simulink model "test_3Lpwm"  (R2025b)
settings: Solver=ode23tb  StartTime=0.0  StopTime=0.2  FixedStep=tc  MaxStep=tc
undefined symbols (not defined in the file or in its folder): dead_time_INV, fPWM_INV, tc, ts_afe
libraries: eePwmGeneratorThreeLevel x1, single_phase_pwm_modulator x1
settings Model: SimulationMode=accelerator  Creator=dbagn  LastModifiedBy=dbagn
settings SolverCC: NumberNewtonIterations=3.0  ZeroCrossControl=DisableAll  AlgebraicLoopSolver=TrustRegion  SolverResetMethod=Robust
settings DataIOCC: ReturnWorkspaceOutputs=off
settings OptimizationCC: ReuseModelBlockBuffer=off
settings DebuggingCC: UnconnectedInputMsg=warning  UnconnectedOutputMsg=warning  UnconnectedLineMsg=warning
settings ModelReferenceCC: EnableRefExpFcnMdlSchedulingChecks=on
settings SFSimCC: CustomCodeUndefinedFunction=ThrowError
settings SFSimCC: SimCustomHeaderCode=|
  | #include "mavgflt.h"
  | #include "mavgflt_simulink.h"
  | #include "bemf_obsv.h"
  | #include "bemf_obsv_simulink.h"
  | #include "bemf_obsv_load_est.h"
  | #include "bemf_obsv_load_est_simulink.h"
  | #include "dqvector_pi.h"
  | #include "dqvector_pi_simulink.h"
  | #include "sv_pwm_simulink.h"
  | #include "sv_pwm.h"
  | #include "first_harmonic_tracker.h"
  | #include "first_harmonic_tracker_simulink.h"
  | #include "dqpll_thyr.h"
  | #include "dqpll_thyr_simulink.h"
  | #include "dqpll_grid.h"
  | #include "dqpll_grid_simulink.h"
settings SFSimCC: SimUserSources=|
  | "mavgflt_simulink.c"
  | "mavgflt.c"
  | "bemf_obsv_simulink.c"
  | "bemf_obsv.c"
  | "bemf_obsv_load_est_simulink.c"
  | "bemf_obsv_load_est.c"
  | "dqvector_pi.c"
  | "dqvector_pi_simulink.c"
  | "sv_pwm_simulink.c"
  | "sv_pwm.c"
  | "first_harmonic_tracker_simulink.c"
  | "first_harmonic_tracker.c"
  | "dqpll_thyr_simulink.c"
  | "dqpll_thyr.c"
  | "dqpll_grid_simulink.c"
  | "dqpll_grid.c"
settings SFSimCC: SimUserIncludeDirs=|
  | include
  | src
settings RTWCC: GPUComputeCapability=3.5  DLArmComputeVersion=19.05

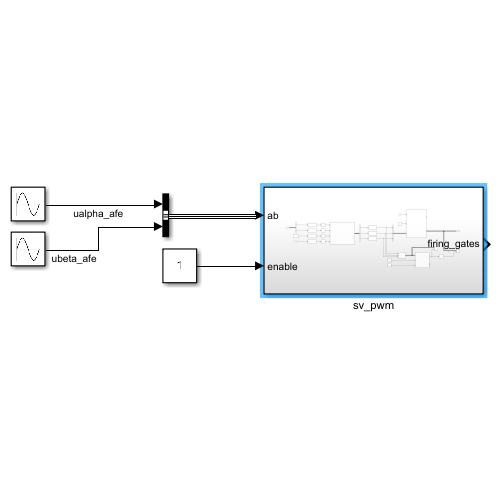
[thumbnail: Simulink's stored preview of the top-level diagram]
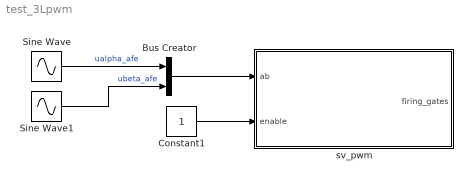
== system test_3Lpwm ==
  Bus Creator : BusCreator  Inputs=2
  Constant1 : Constant
  Sine Wave : Sin  Amplitude=sqrt(3)/2  Frequency=2*pi*50  Phase=-pi/2  SampleTime=0
  Sine Wave1 : Sin  Amplitude=sqrt(3)/2  Frequency=2*pi*50  SampleTime=0
  sv_pwm : Subsystem
  wires:
  Constant1/1 -> sv_pwm/2(enable)
  Bus Creator/1 -> sv_pwm/1(ab)
  Sine Wave/1 -> Bus Creator/1  "ualpha_afe"
  Sine Wave1/1 -> Bus Creator/2  "ubeta_afe"

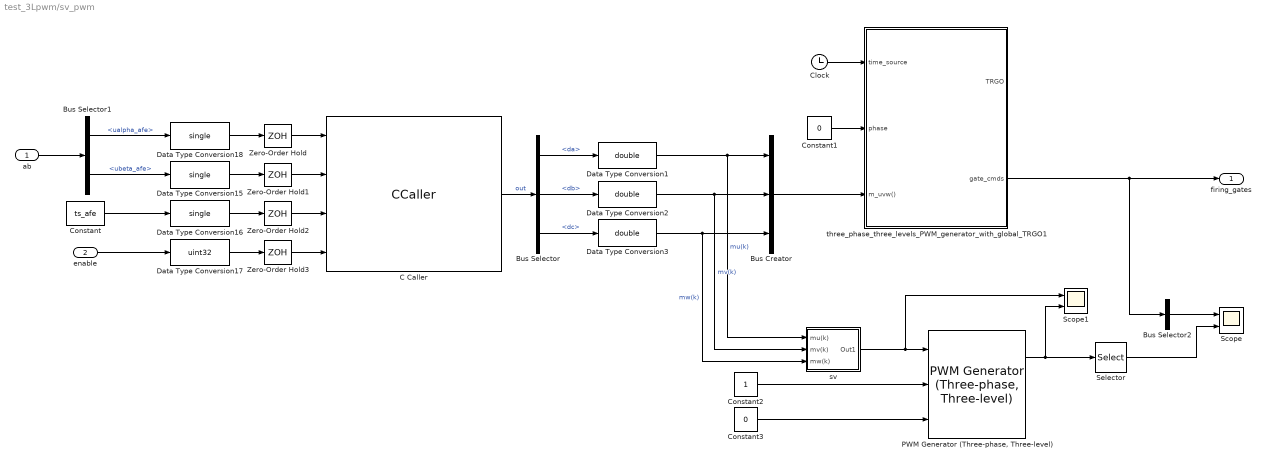
== system test_3Lpwm/sv_pwm ==
  ab : Inport
  enable : Inport  Port=2
  Bus Creator : BusCreator  Inputs=3
  Bus Selector : BusSelector  OutputSignals=da,db,dc
  Bus Selector1 : BusSelector  OutputSignals=ualpha_afe,ubeta_afe
  Bus Selector2 : BusSelector  OutputSignals=gate_cmds_phu  OutputAsBus=on
  C Caller : CCaller  FunctionName=sv_pwm_process_simulink  PortSpecificationStruct="%)30     .    V @   8    (     @         %    \"     4    !     0         %  0 \"0    $    _    07)G3F%M90  4&]R=$YA;64 4V-O<&4     26YD97@     5'EP90      4VEZ90      27-';&]B86P   X    P    !@    @    $          4    (     0    ,    !         !   P!O=70 #@   #     &    \"     0         !0    @    !     P    $         $  # &]U=  .    .     8    (    !          %    \"     $    &     0         0   ...(+2669 chars)"  SampleTime=ts_afe
  Clock : Clock
  Constant : Constant  Value=ts_afe
  Constant1 : Constant  Value=0
  Constant2 : Constant
  Constant3 : Constant  Value=0
  Data Type Conversion1 : DataTypeConversion  OutDataTypeStr=double  SaturateOnIntegerOverflow=off  RndMeth=Floor
  Data Type Conversion15 : DataTypeConversion  OutDataTypeStr=single  SaturateOnIntegerOverflow=off  RndMeth=Floor
  Data Type Conversion16 : DataTypeConversion  OutDataTypeStr=single  SaturateOnIntegerOverflow=off  RndMeth=Floor
  Data Type Conversion17 : DataTypeConversion  OutDataTypeStr=uint32  SaturateOnIntegerOverflow=off  RndMeth=Floor
  Data Type Conversion18 : DataTypeConversion  OutDataTypeStr=single  SaturateOnIntegerOverflow=off  RndMeth=Floor
  Data Type Conversion2 : DataTypeConversion  OutDataTypeStr=double  SaturateOnIntegerOverflow=off  RndMeth=Floor
  Data Type Conversion3 : DataTypeConversion  OutDataTypeStr=double  SaturateOnIntegerOverflow=off  RndMeth=Floor
  "PWM Generator (Three-phase, Three-level)" : eePwmGeneratorThreeLevel/PWM Generator (Three-phase, Three-level)  CPWMMode=SPWM: sinusoidal PWM  fsw=1e3  Ts=5e-5
      settings: SamplingMode=Natural
      settings: LibrarySourceBlock=|
      | ee_sl_lib/Pulse Width
      | Modulation/PWM Generator
      | (Three-phase, Three-level)
  Scope : Scope  NumInputPorts=2
      settings: ActiveDisplayYMinimum=-13.125  ActiveDisplayYMaximum=18.125  DataLoggingVariableName=ScopeData6
  Scope1 : Scope  NumInputPorts=2
      settings: ActiveDisplayYMinimum=-2.2498929426074028  ActiveDisplayYMaximum=0.24989300221204752
  Selector : Selector  InputPortWidth=12  IndexOptions=Index vector (dialog)  Indices=[1 2 3 4]  OutputSizes=1
  Zero-Order Hold{,1..3} (4 alike) : ZeroOrderHold  SampleTime=ts_afe
  sv : Subsystem
  three_phase_three_levels_PWM_generator_with_global_TRGO1 : Subsystem  mask{f=fPWM_INV, m_up=1, m_low=-1, dead_time=dead_time_INV, pos_cmd_gate=15, neg_cmd_gate=-10, polarity=1, tc=tc, double_sampling=1}
      mask prompts: f "Frequency (Hz)"; m_up "Max Input Modulation Value"; m_low "Min Input Modulation Value"; dead_time "Dead Time (s)"; pos_cmd_gate "Positive Gate Voltage (V)"; neg_cmd_gate "Negative Gate Voltage (V)"; polarity "Polarity (pu)"; tc "Sampling time"; double_sampling "double TRGO update"
  firing_gates : Outport
  wires:
  Zero-Order Hold2/1 -> C Caller/3
  Constant/1 -> Data Type Conversion16/1
  Data Type Conversion18/1 -> Zero-Order Hold/1
  enable/1 -> Data Type Conversion17/1
  Data Type Conversion16/1 -> Zero-Order Hold2/1
  Data Type Conversion17/1 -> Zero-Order Hold3/1
  Zero-Order Hold3/1 -> C Caller/4
  Data Type Conversion15/1 -> Zero-Order Hold1/1
  three_phase_three_levels_PWM_generator_with_global_TRGO1/2(gate_cmds) -> Bus Selector2/1, firing_gates/1
  Bus Selector1/1 -> Data Type Conversion18/1  "<ualpha_afe>"
  Bus Selector1/2 -> Data Type Conversion15/1  "<ubeta_afe>"
  Data Type Conversion3/1 -> sv/3(mw(k)), Bus Creator/3  "mw(k)"
  Data Type Conversion2/1 -> sv/2(mv(k)), Bus Creator/2  "mv(k)"
  Data Type Conversion1/1 -> sv/1(mu(k)), Bus Creator/1  "mu(k)"
  ab/1 -> Bus Selector1/1
  Zero-Order Hold/1 -> C Caller/1
  Zero-Order Hold1/1 -> C Caller/2
  C Caller/1 -> Bus Selector/1  "out"
  Bus Selector/1 -> Data Type Conversion1/1  "<da>"
  Bus Selector/2 -> Data Type Conversion2/1  "<db>"
  Bus Selector/3 -> Data Type Conversion3/1  "<dc>"
  Clock/1 -> three_phase_three_levels_PWM_generator_with_global_TRGO1/1(time_source)
  Bus Creator/1 -> three_phase_three_levels_PWM_generator_with_global_TRGO1/3(m_uvw())
  Constant1/1 -> three_phase_three_levels_PWM_generator_with_global_TRGO1/2(phase)
  Bus Selector2/1 -> Scope/1
  Constant2/1 -> "PWM Generator (Three-phase, Three-level)"/2
  Constant3/1 -> "PWM Generator (Three-phase, Three-level)"/3
  "PWM Generator (Three-phase, Three-level)"/1 -> Scope1/2, Selector/1
  Selector/1 -> Scope/2
  sv/1(Out1) -> Scope1/1, "PWM Generator (Three-phase, Three-level)"/1

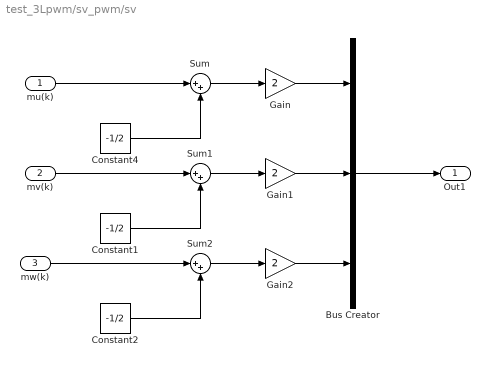
== system test_3Lpwm/sv_pwm/sv ==
  mu(k) : Inport
  mv(k) : Inport  Port=2
  mw(k) : Inport  Port=3
  Bus Creator : BusCreator  Inputs=3
  Constant1 : Constant  Value=-1/2
  Constant2 : Constant  Value=-1/2
  Constant4 : Constant  Value=-1/2
  Gain : Gain  Gain=2
  Gain1 : Gain  Gain=2
  Gain2 : Gain  Gain=2
  Sum : Sum  Inputs=|++
  Sum1 : Sum  Inputs=|++
  Sum2 : Sum  Inputs=|++
  Out1 : Outport
  wires:
  Sum/1 -> Gain/1
  mu(k)/1 -> Sum/1
  Constant4/1 -> Sum/2
  Gain/1 -> Bus Creator/1
  Bus Creator/1 -> Out1/1
  Constant1/1 -> Sum1/2
  Sum1/1 -> Gain1/1
  Gain1/1 -> Bus Creator/2
  mv(k)/1 -> Sum1/1
  mw(k)/1 -> Sum2/1
  Sum2/1 -> Gain2/1
  Constant2/1 -> Sum2/2
  Gain2/1 -> Bus Creator/3

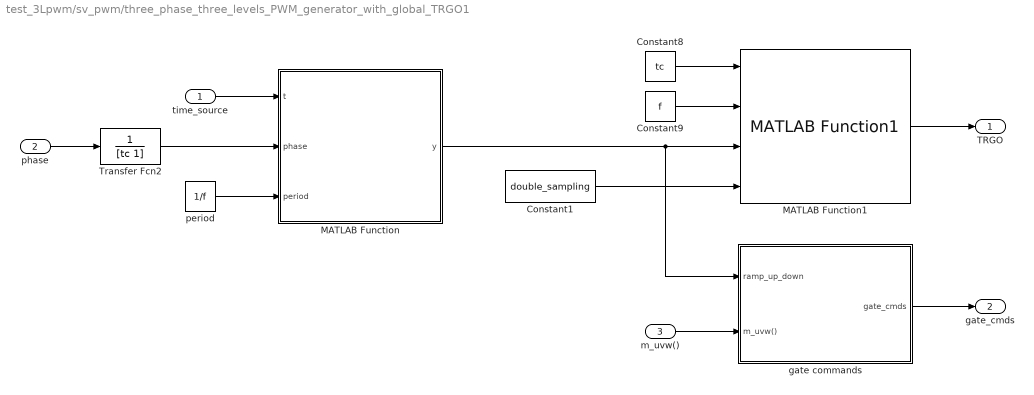
== system test_3Lpwm/sv_pwm/three_phase_three_levels_PWM_generator_with_global_TRGO1 ==
  time_source : Inport
  phase : Inport  Port=2
  m_uvw() : Inport  Port=3
  Constant1 : Constant  Value=double_sampling
  Constant8 : Constant  Value=tc
  Constant9 : Constant  Value=f
  MATLAB Function : MATLAB Function  TreatAsAtomicUnit=on  SystemSampleTime=tc
  MATLAB Function1 : single_phase_pwm_modulator/Single phase two level PWM generator with global TRGO/MATLAB Function1  SystemSampleTime=tc  VariantActivationTime=update diagram  EmptyChoice=off  PassThrough=off  PassThroughVariantControl=(default)  EmptyChoiceVariantControl=(default)  AllowFlexibleInterface=on  Latency=0  AutoFrameSizeCalculation=off
  Transfer Fcn2 : TransferFcn  Denominator=[tc 1]
  gate commands : Subsystem
  period : Constant  Value=1/f
  TRGO : Outport
  gate_cmds : Outport  Port=2
  wires:
  Transfer Fcn2/1 -> MATLAB Function/2(phase)
  Constant1/1 -> MATLAB Function1/4
  time_source/1 -> MATLAB Function/1(t)
  gate commands/1(gate_cmds) -> gate_cmds/1
  m_uvw()/1 -> gate commands/2(m_uvw())
  Constant9/1 -> MATLAB Function1/2
  Constant8/1 -> MATLAB Function1/1
  MATLAB Function1/1 -> TRGO/1
  MATLAB Function/1(y) -> MATLAB Function1/3, gate commands/1(ramp_up_down)
  phase/1 -> Transfer Fcn2/1
  period/1 -> MATLAB Function/3(period)

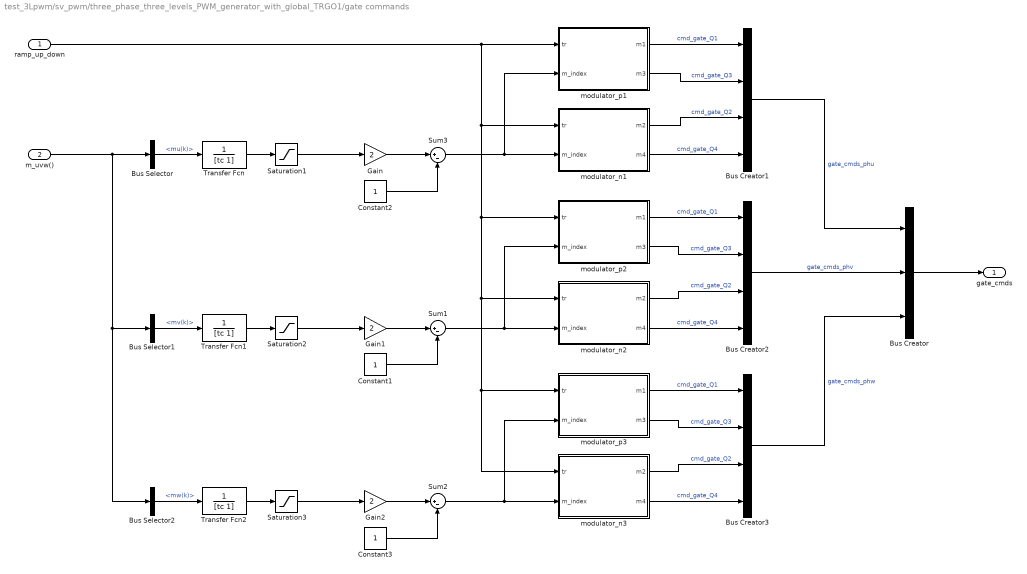
== system test_3Lpwm/sv_pwm/three_phase_three_levels_PWM_generator_with_global_TRGO1/gate commands ==
  ramp_up_down : Inport
  m_uvw() : Inport  Port=2
  Bus Creator : BusCreator  Inputs=3
  Bus Creator1 : BusCreator  Inputs=4
  Bus Creator2 : BusCreator  Inputs=4
  Bus Creator3 : BusCreator  Inputs=4
  Bus Selector : BusSelector  OutputSignals=mu(k)
  Bus Selector1 : BusSelector  OutputSignals=mv(k)
  Bus Selector2 : BusSelector  OutputSignals=mw(k)
  Constant1 : Constant
  Constant2 : Constant
  Constant3 : Constant
  Gain : Gain  Gain=2
  Gain1 : Gain  Gain=2
  Gain2 : Gain  Gain=2
  Saturation1 : Saturate  UpperLimit=m_up  LowerLimit=m_low
  Saturation2 : Saturate  UpperLimit=m_up  LowerLimit=m_low
  Saturation3 : Saturate  UpperLimit=m_up  LowerLimit=m_low
  Sum1 : Sum  Inputs=|+-
  Sum2 : Sum  Inputs=|+-
  Sum3 : Sum  Inputs=|+-
  Transfer Fcn : TransferFcn  Denominator=[tc 1]
  Transfer Fcn1 : TransferFcn  Denominator=[tc 1]
  Transfer Fcn2 : TransferFcn  Denominator=[tc 1]
  modulator_n1 : Subsystem
  modulator_n2 : Subsystem
  modulator_n3 : Subsystem
  modulator_p1 : Subsystem
  modulator_p2 : Subsystem
  modulator_p3 : Subsystem
  gate_cmds : Outport
  wires:
  Transfer Fcn2/1 -> Saturation3/1
  Transfer Fcn1/1 -> Saturation2/1
  Transfer Fcn/1 -> Saturation1/1
  Bus Selector/1 -> Transfer Fcn/1  "<mu(k)>"
  Bus Selector2/1 -> Transfer Fcn2/1  "<mw(k)>"
  Bus Selector1/1 -> Transfer Fcn1/1  "<mv(k)>"
  Bus Creator/1 -> gate_cmds/1
  m_uvw()/1 -> Bus Selector/1, Bus Selector1/1, Bus Selector2/1
  Gain/1 -> Sum3/1
  Sum3/1 -> modulator_p1/2(m_index), modulator_n1/2(m_index)
  Constant2/1 -> Sum3/2
  Saturation1/1 -> Gain/1
  modulator_p1/1(m1) -> Bus Creator1/1  "cmd_gate_Q1"
  modulator_p1/2(m3) -> Bus Creator1/2  "cmd_gate_Q3"
  modulator_n1/1(m2) -> Bus Creator1/3  "cmd_gate_Q2"
  modulator_n1/2(m4) -> Bus Creator1/4  "cmd_gate_Q4"
  Bus Creator1/1 -> Bus Creator/1  "gate_cmds_phu"
  Bus Creator2/1 -> Bus Creator/2  "gate_cmds_phv"
  modulator_n2/2(m4) -> Bus Creator2/4  "cmd_gate_Q4"
  modulator_n2/1(m2) -> Bus Creator2/3  "cmd_gate_Q2"
  modulator_p2/2(m3) -> Bus Creator2/2  "cmd_gate_Q3"
  modulator_p2/1(m1) -> Bus Creator2/1  "cmd_gate_Q1"
  ramp_up_down/1 -> modulator_n2/1(tr), modulator_p3/1(tr), modulator_n3/1(tr), modulator_p2/1(tr), modulator_n1/1(tr), modulator_p1/1(tr)
  modulator_p3/1(m1) -> Bus Creator3/1  "cmd_gate_Q1"
  modulator_p3/2(m3) -> Bus Creator3/2  "cmd_gate_Q3"
  modulator_n3/1(m2) -> Bus Creator3/3  "cmd_gate_Q2"
  modulator_n3/2(m4) -> Bus Creator3/4  "cmd_gate_Q4"
  Bus Creator3/1 -> Bus Creator/3  "gate_cmds_phw"
  Constant1/1 -> Sum1/2
  Gain1/1 -> Sum1/1
  Saturation2/1 -> Gain1/1
  Sum1/1 -> modulator_p2/2(m_index), modulator_n2/2(m_index)
  Sum2/1 -> modulator_n3/2(m_index), modulator_p3/2(m_index)
  Saturation3/1 -> Gain2/1
  Gain2/1 -> Sum2/1
  Constant3/1 -> Sum2/2

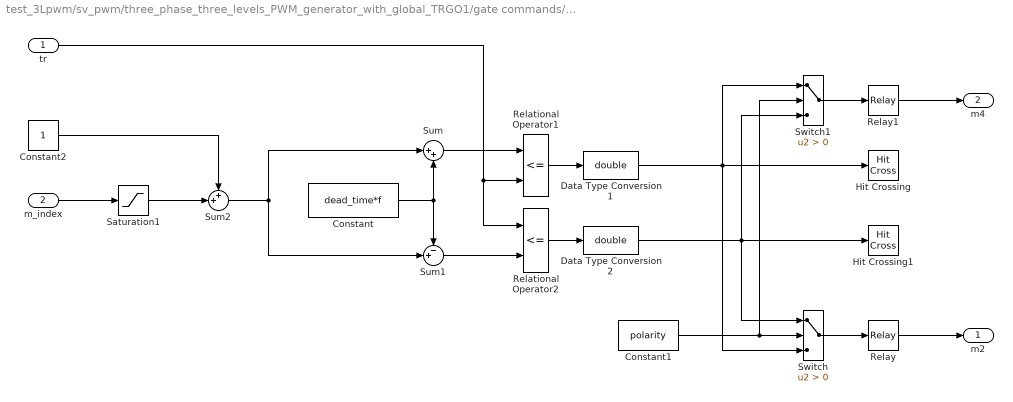
== system test_3Lpwm/sv_pwm/three_phase_three_levels_PWM_generator_with_global_TRGO1/gate commands/modulator_n1 ==
  tr : Inport
  m_index : Inport  Port=2
  Constant : Constant  Value=dead_time*f
  Constant1 : Constant  Value=polarity
  Constant2 : Constant
  Data Type Conversion1 : DataTypeConversion  OutDataTypeStr=double
  Data Type Conversion2 : DataTypeConversion  OutDataTypeStr=double
  Hit Crossing : HitCross  ShowOutputPort=off
  Hit Crossing1 : HitCross  ShowOutputPort=off
  Relational Operator1 : RelationalOperator  Operator=<=  InputSameDT=off
  Relational Operator2 : RelationalOperator  Operator=<=  InputSameDT=off
  Relay : Relay  OnOutputValue=pos_cmd_gate  OffOutputValue=neg_cmd_gate
  Relay1 : Relay  OnOutputValue=pos_cmd_gate  OffOutputValue=neg_cmd_gate
  Saturation1 : Saturate  UpperLimit=0  LowerLimit=m_low
  Sum : Sum  Inputs=|++  SaturateOnIntegerOverflow=on
  Sum1 : Sum  Inputs=-+|  SaturateOnIntegerOverflow=on
  Sum2 : Sum  Inputs=++|  SaturateOnIntegerOverflow=on
  Switch : Switch  Criteria=u2 > Threshold  SaturateOnIntegerOverflow=off  InputSameDT=off
  Switch1 : Switch  Criteria=u2 > Threshold  SaturateOnIntegerOverflow=off  InputSameDT=off
  m2 : Outport
  m4 : Outport  Port=2
  wires:
  Relay1/1 -> m4/1
  Relay/1 -> m2/1
  Switch1/1 -> Relay1/1
  tr/1 -> Relational Operator1/2, Relational Operator2/1
  Sum/1 -> Relational Operator1/1
  Constant/1 -> Sum1/1, Sum/2
  Switch/1 -> Relay/1
  Data Type Conversion2/1 -> Hit Crossing1/1, Switch1/3, Switch/1
  Constant1/1 -> Switch/2, Switch1/2
  Sum1/1 -> Relational Operator2/2
  Data Type Conversion1/1 -> Switch1/1, Switch/3, Hit Crossing/1
  Relational Operator1/1 -> Data Type Conversion1/1
  Relational Operator2/1 -> Data Type Conversion2/1
  m_index/1 -> Saturation1/1
  Saturation1/1 -> Sum2/2
  Sum2/1 -> Sum1/2, Sum/1
  Constant2/1 -> Sum2/1

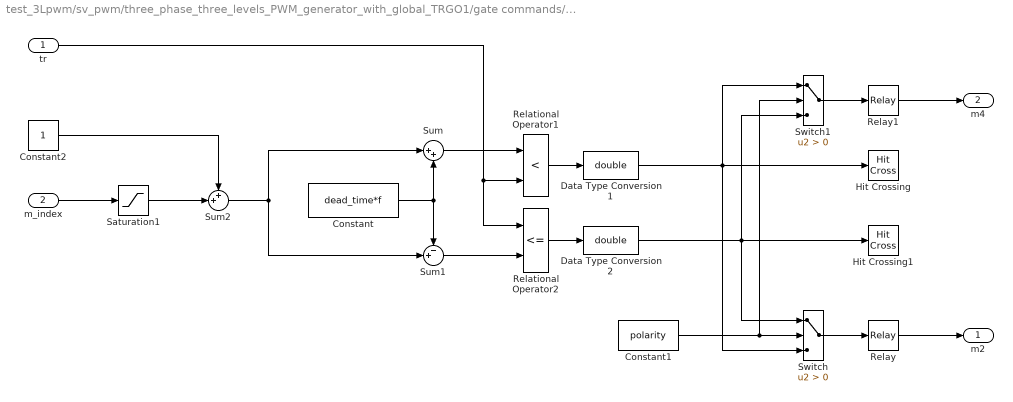
== system test_3Lpwm/sv_pwm/three_phase_three_levels_PWM_generator_with_global_TRGO1/gate commands/modulator_n2 ==
  tr : Inport
  m_index : Inport  Port=2
  Constant : Constant  Value=dead_time*f
  Constant1 : Constant  Value=polarity
  Constant2 : Constant
  Data Type Conversion1 : DataTypeConversion  OutDataTypeStr=double
  Data Type Conversion2 : DataTypeConversion  OutDataTypeStr=double
  Hit Crossing : HitCross  ShowOutputPort=off
  Hit Crossing1 : HitCross  ShowOutputPort=off
  Relational Operator1 : RelationalOperator  Operator=<  InputSameDT=off
  Relational Operator2 : RelationalOperator  Operator=<=  InputSameDT=off
  Relay : Relay  OnOutputValue=pos_cmd_gate  OffOutputValue=neg_cmd_gate
  Relay1 : Relay  OnOutputValue=pos_cmd_gate  OffOutputValue=neg_cmd_gate
  Saturation1 : Saturate  UpperLimit=0  LowerLimit=m_low
  Sum : Sum  Inputs=|++  SaturateOnIntegerOverflow=on
  Sum1 : Sum  Inputs=-+|  SaturateOnIntegerOverflow=on
  Sum2 : Sum  Inputs=++|  SaturateOnIntegerOverflow=on
  Switch : Switch  Criteria=u2 > Threshold  SaturateOnIntegerOverflow=off  InputSameDT=off
  Switch1 : Switch  Criteria=u2 > Threshold  SaturateOnIntegerOverflow=off  InputSameDT=off
  m2 : Outport
  m4 : Outport  Port=2
  wires:
  Constant2/1 -> Sum2/1
  Sum2/1 -> Sum/1, Sum1/2
  Saturation1/1 -> Sum2/2
  m_index/1 -> Saturation1/1
  Relational Operator2/1 -> Data Type Conversion2/1
  Relational Operator1/1 -> Data Type Conversion1/1
  Data Type Conversion1/1 -> Hit Crossing/1, Switch/3, Switch1/1
  Sum1/1 -> Relational Operator2/2
  Constant1/1 -> Switch1/2, Switch/2
  Data Type Conversion2/1 -> Switch/1, Switch1/3, Hit Crossing1/1
  Switch/1 -> Relay/1
  Constant/1 -> Sum/2, Sum1/1
  Sum/1 -> Relational Operator1/1
  tr/1 -> Relational Operator2/1, Relational Operator1/2
  Switch1/1 -> Relay1/1
  Relay/1 -> m2/1
  Relay1/1 -> m4/1

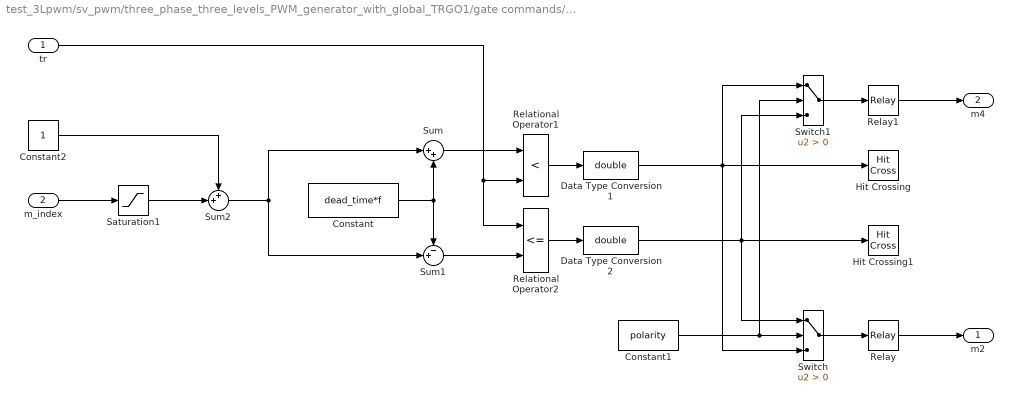
== system test_3Lpwm/sv_pwm/three_phase_three_levels_PWM_generator_with_global_TRGO1/gate commands/modulator_n3 ==
  tr : Inport
  m_index : Inport  Port=2
  Constant : Constant  Value=dead_time*f
  Constant1 : Constant  Value=polarity
  Constant2 : Constant
  Data Type Conversion1 : DataTypeConversion  OutDataTypeStr=double
  Data Type Conversion2 : DataTypeConversion  OutDataTypeStr=double
  Hit Crossing : HitCross  ShowOutputPort=off
  Hit Crossing1 : HitCross  ShowOutputPort=off
  Relational Operator1 : RelationalOperator  Operator=<  InputSameDT=off
  Relational Operator2 : RelationalOperator  Operator=<=  InputSameDT=off
  Relay : Relay  OnOutputValue=pos_cmd_gate  OffOutputValue=neg_cmd_gate
  Relay1 : Relay  OnOutputValue=pos_cmd_gate  OffOutputValue=neg_cmd_gate
  Saturation1 : Saturate  UpperLimit=0  LowerLimit=m_low
  Sum : Sum  Inputs=|++  SaturateOnIntegerOverflow=on
  Sum1 : Sum  Inputs=-+|  SaturateOnIntegerOverflow=on
  Sum2 : Sum  Inputs=++|  SaturateOnIntegerOverflow=on
  Switch : Switch  Criteria=u2 > Threshold  SaturateOnIntegerOverflow=off  InputSameDT=off
  Switch1 : Switch  Criteria=u2 > Threshold  SaturateOnIntegerOverflow=off  InputSameDT=off
  m2 : Outport
  m4 : Outport  Port=2
  wires:
  Relay1/1 -> m4/1
  Relay/1 -> m2/1
  Switch1/1 -> Relay1/1
  tr/1 -> Relational Operator1/2, Relational Operator2/1
  Sum/1 -> Relational Operator1/1
  Constant/1 -> Sum1/1, Sum/2
  Switch/1 -> Relay/1
  Data Type Conversion2/1 -> Hit Crossing1/1, Switch1/3, Switch/1
  Constant1/1 -> Switch/2, Switch1/2
  Sum1/1 -> Relational Operator2/2
  Data Type Conversion1/1 -> Switch1/1, Switch/3, Hit Crossing/1
  Relational Operator1/1 -> Data Type Conversion1/1
  Relational Operator2/1 -> Data Type Conversion2/1
  m_index/1 -> Saturation1/1
  Saturation1/1 -> Sum2/2
  Sum2/1 -> Sum1/2, Sum/1
  Constant2/1 -> Sum2/1

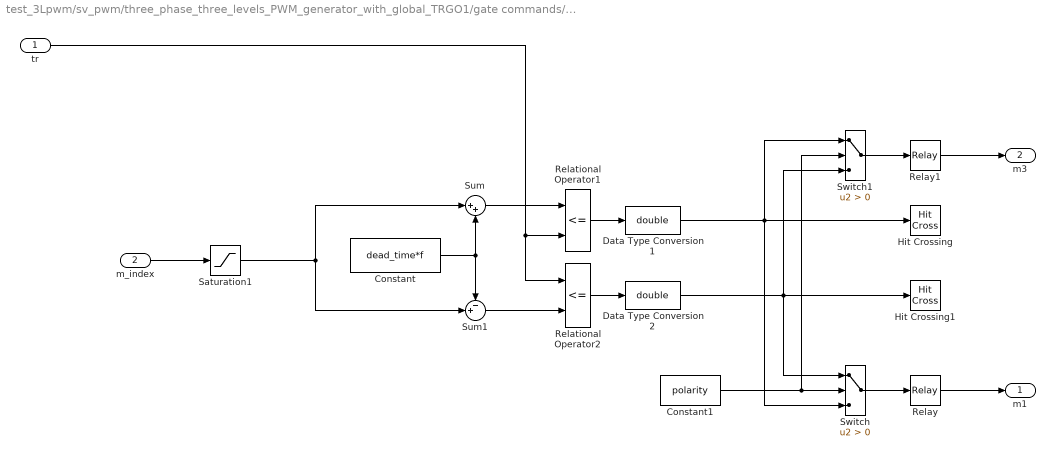
== system test_3Lpwm/sv_pwm/three_phase_three_levels_PWM_generator_with_global_TRGO1/gate commands/modulator_p1 ==
  tr : Inport
  m_index : Inport  Port=2
  Constant : Constant  Value=dead_time*f
  Constant1 : Constant  Value=polarity
  Data Type Conversion1 : DataTypeConversion  OutDataTypeStr=double
  Data Type Conversion2 : DataTypeConversion  OutDataTypeStr=double
  Hit Crossing : HitCross  ShowOutputPort=off
  Hit Crossing1 : HitCross  ShowOutputPort=off
  Relational Operator1 : RelationalOperator  Operator=<=  InputSameDT=off
  Relational Operator2 : RelationalOperator  Operator=<=  InputSameDT=off
  Relay : Relay  OnSwitchValue=2*eps  OnOutputValue=pos_cmd_gate  OffOutputValue=neg_cmd_gate
  Relay1 : Relay  OnOutputValue=pos_cmd_gate  OffOutputValue=neg_cmd_gate
  Saturation1 : Saturate  UpperLimit=m_up  LowerLimit=0
  Sum : Sum  Inputs=|++  SaturateOnIntegerOverflow=on
  Sum1 : Sum  Inputs=-+|  SaturateOnIntegerOverflow=on
  Switch : Switch  Criteria=u2 > Threshold  SaturateOnIntegerOverflow=off  InputSameDT=off
  Switch1 : Switch  Criteria=u2 > Threshold  SaturateOnIntegerOverflow=off  InputSameDT=off
  m1 : Outport
  m3 : Outport  Port=2
  wires:
  m_index/1 -> Saturation1/1
  Relational Operator2/1 -> Data Type Conversion2/1
  Relational Operator1/1 -> Data Type Conversion1/1
  Data Type Conversion1/1 -> Hit Crossing/1, Switch/3, Switch1/1
  Sum1/1 -> Relational Operator2/2
  Saturation1/1 -> Sum/1, Sum1/2
  Constant1/1 -> Switch1/2, Switch/2
  Data Type Conversion2/1 -> Switch/1, Switch1/3, Hit Crossing1/1
  Switch/1 -> Relay/1
  Constant/1 -> Sum/2, Sum1/1
  Sum/1 -> Relational Operator1/1
  tr/1 -> Relational Operator2/1, Relational Operator1/2
  Switch1/1 -> Relay1/1
  Relay/1 -> m1/1
  Relay1/1 -> m3/1

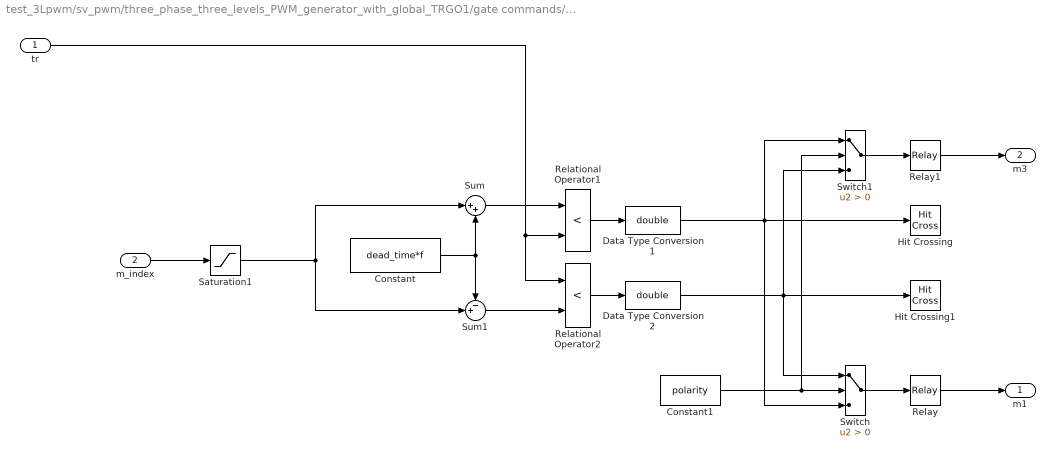
== system test_3Lpwm/sv_pwm/three_phase_three_levels_PWM_generator_with_global_TRGO1/gate commands/modulator_p2 ==
  tr : Inport
  m_index : Inport  Port=2
  Constant : Constant  Value=dead_time*f
  Constant1 : Constant  Value=polarity
  Data Type Conversion1 : DataTypeConversion  OutDataTypeStr=double
  Data Type Conversion2 : DataTypeConversion  OutDataTypeStr=double
  Hit Crossing : HitCross  ShowOutputPort=off
  Hit Crossing1 : HitCross  ShowOutputPort=off
  Relational Operator1 : RelationalOperator  Operator=<  InputSameDT=off
  Relational Operator2 : RelationalOperator  Operator=<  InputSameDT=off
  Relay : Relay  OnSwitchValue=2*eps  OnOutputValue=pos_cmd_gate  OffOutputValue=neg_cmd_gate
  Relay1 : Relay  OnOutputValue=pos_cmd_gate  OffOutputValue=neg_cmd_gate
  Saturation1 : Saturate  UpperLimit=m_up  LowerLimit=0
  Sum : Sum  Inputs=|++  SaturateOnIntegerOverflow=on
  Sum1 : Sum  Inputs=-+|  SaturateOnIntegerOverflow=on
  Switch : Switch  Criteria=u2 > Threshold  SaturateOnIntegerOverflow=off  InputSameDT=off
  Switch1 : Switch  Criteria=u2 > Threshold  SaturateOnIntegerOverflow=off  InputSameDT=off
  m1 : Outport
  m3 : Outport  Port=2
  wires:
  Relay1/1 -> m3/1
  Relay/1 -> m1/1
  Switch1/1 -> Relay1/1
  tr/1 -> Relational Operator1/2, Relational Operator2/1
  Sum/1 -> Relational Operator1/1
  Constant/1 -> Sum1/1, Sum/2
  Switch/1 -> Relay/1
  Data Type Conversion2/1 -> Hit Crossing1/1, Switch1/3, Switch/1
  Constant1/1 -> Switch/2, Switch1/2
  Saturation1/1 -> Sum1/2, Sum/1
  Sum1/1 -> Relational Operator2/2
  Data Type Conversion1/1 -> Switch1/1, Switch/3, Hit Crossing/1
  Relational Operator1/1 -> Data Type Conversion1/1
  Relational Operator2/1 -> Data Type Conversion2/1
  m_index/1 -> Saturation1/1

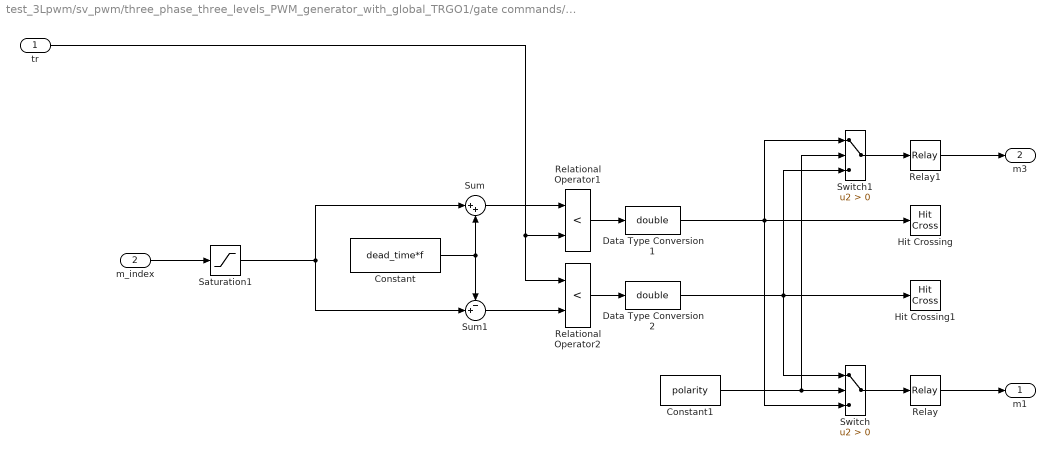
== system test_3Lpwm/sv_pwm/three_phase_three_levels_PWM_generator_with_global_TRGO1/gate commands/modulator_p3 ==
  tr : Inport
  m_index : Inport  Port=2
  Constant : Constant  Value=dead_time*f
  Constant1 : Constant  Value=polarity
  Data Type Conversion1 : DataTypeConversion  OutDataTypeStr=double
  Data Type Conversion2 : DataTypeConversion  OutDataTypeStr=double
  Hit Crossing : HitCross  ShowOutputPort=off
  Hit Crossing1 : HitCross  ShowOutputPort=off
  Relational Operator1 : RelationalOperator  Operator=<  InputSameDT=off
  Relational Operator2 : RelationalOperator  Operator=<  InputSameDT=off
  Relay : Relay  OnSwitchValue=2*eps  OnOutputValue=pos_cmd_gate  OffOutputValue=neg_cmd_gate
  Relay1 : Relay  OnOutputValue=pos_cmd_gate  OffOutputValue=neg_cmd_gate
  Saturation1 : Saturate  UpperLimit=m_up  LowerLimit=0
  Sum : Sum  Inputs=|++  SaturateOnIntegerOverflow=on
  Sum1 : Sum  Inputs=-+|  SaturateOnIntegerOverflow=on
  Switch : Switch  Criteria=u2 > Threshold  SaturateOnIntegerOverflow=off  InputSameDT=off
  Switch1 : Switch  Criteria=u2 > Threshold  SaturateOnIntegerOverflow=off  InputSameDT=off
  m1 : Outport
  m3 : Outport  Port=2
  wires:
  m_index/1 -> Saturation1/1
  Relational Operator2/1 -> Data Type Conversion2/1
  Relational Operator1/1 -> Data Type Conversion1/1
  Data Type Conversion1/1 -> Hit Crossing/1, Switch/3, Switch1/1
  Sum1/1 -> Relational Operator2/2
  Saturation1/1 -> Sum/1, Sum1/2
  Constant1/1 -> Switch1/2, Switch/2
  Data Type Conversion2/1 -> Switch/1, Switch1/3, Hit Crossing1/1
  Switch/1 -> Relay/1
  Constant/1 -> Sum/2, Sum1/1
  Sum/1 -> Relational Operator1/1
  tr/1 -> Relational Operator2/1, Relational Operator1/2
  Switch1/1 -> Relay1/1
  Relay/1 -> m1/1
  Relay1/1 -> m3/1

== matlab function test_3Lpwm/sv_pwm/three_phase_three_levels_PWM_generator_with_global_TRGO1/MATLAB Function ==
  data: t input; y output; phase input; period input
function y = ramp_up_down(t,phase,period)
x = sin(2*pi/period*t - phase -pi/2);
y = asin(x)/pi + 1/2;
